simulink model "adaptive_dcmotor_2nd_sim"  (R2025b)
settings: Solver=FixedStepDiscrete  StartTime=0.0  StopTime=8  FixedStep=0.002  RelTol=1e-3
model workspace (MAT data in the model file):
  refProfile = [0 0.002 0.004 0.006 0.008 0.01 0.012 0.014 0.016 0.018 0.02 0.022 ... (8002 elements, 4001x2)]
(part 1 of 2)
settings Model: Creator=Lenard  LastModifiedBy=Lenard

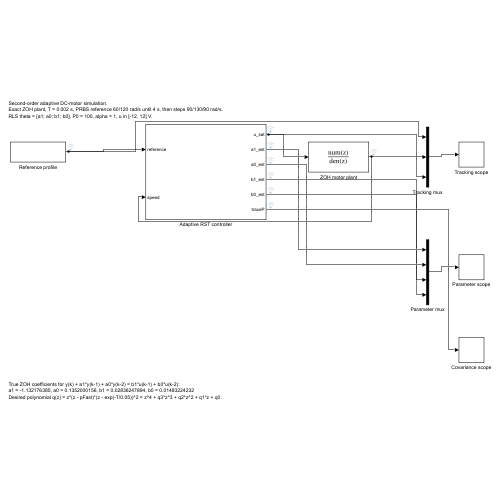
[thumbnail: Simulink's stored preview of the top-level diagram]
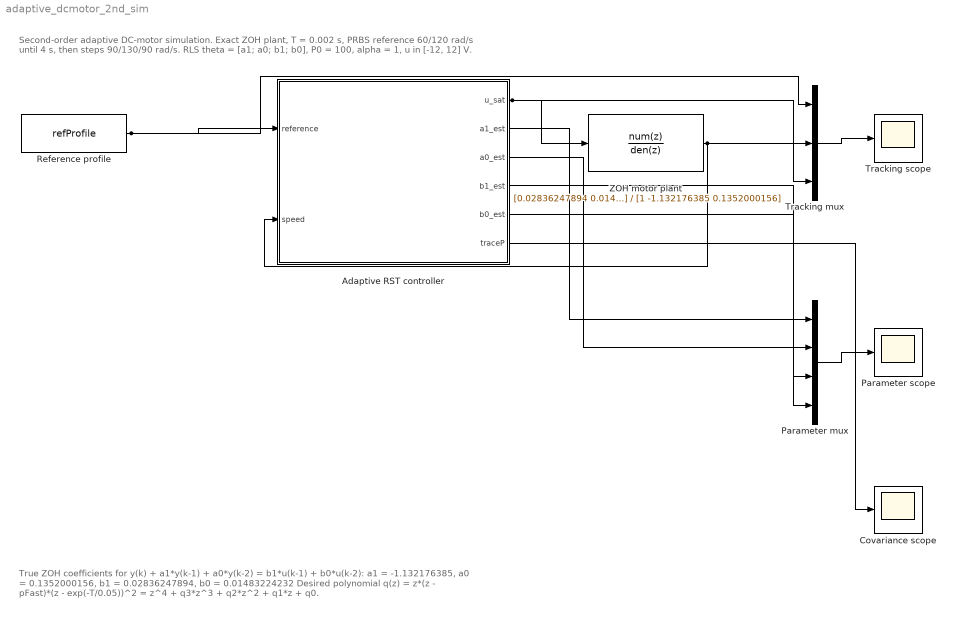
== system adaptive_dcmotor_2nd_sim ==
  note: Second-order adaptive DC-motor simulation.
      | Exact ZOH plant, T = 0.002 s, PRBS reference 60/120 rad/s until 4 s, then steps 90/130/90 rad/s.
      | RLS theta = [a1; a0; b1; b0], P0 = 100, alpha = 1, u in [-12, 12] V.
  note: True ZOH coefficients for y(k) + a1*y(k-1) + a0*y(k-2) = b1*u(k-1) + b0*u(k-2):
      | a1 = -1.132176385, a0 = 0.1352000156, b1 = 0.02836247894, b0 = 0.01483224232
      | Desired polynomial q(z) = z*(z - pFast)*(z - exp(-T/0.05))^2 = z^4 + q3*z^3 + q2*z^2 + q1*z + q0.
  Adaptive RST controller : Subsystem
  Covariance scope : Scope
  Parameter mux : Mux
  Parameter scope : Scope
  Reference profile : FromWorkspace  VariableName=refProfile  SampleTime=0.002  Interpolate=off  OutputAfterFinalValue=Holding final value
  Tracking mux : Mux  Inputs=3
  Tracking scope : Scope
  ZOH motor plant : DiscreteTransferFcn  Numerator=[0.02836247894 0.01483224232]  Denominator=[1 -1.132176385 0.1352000156]  SampleTime=0.002
  wires:
  Reference profile/1 -> Adaptive RST controller/1(reference), Tracking mux/1
  Adaptive RST controller/1(u_sat) -> ZOH motor plant/1, Tracking mux/3
  ZOH motor plant/1 -> Adaptive RST controller/2(speed), Tracking mux/2
  Tracking mux/1 -> Tracking scope/1
  Adaptive RST controller/2(a1_est) -> Parameter mux/1
  Adaptive RST controller/3(a0_est) -> Parameter mux/2
  Adaptive RST controller/4(b1_est) -> Parameter mux/3
  Adaptive RST controller/5(b0_est) -> Parameter mux/4
  Parameter mux/1 -> Parameter scope/1
  Adaptive RST controller/6(traceP) -> Covariance scope/1

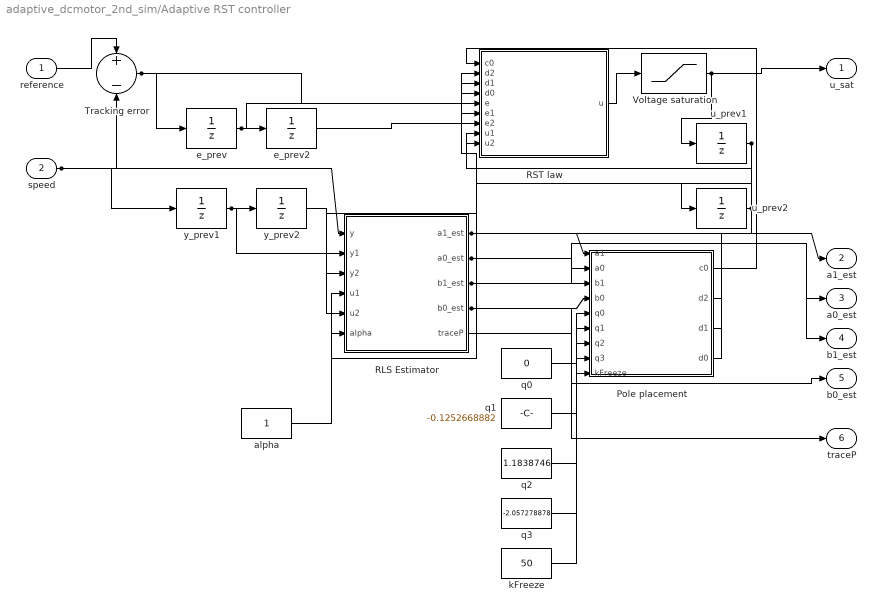
== system adaptive_dcmotor_2nd_sim/Adaptive RST controller ==
  reference : Inport
  speed : Inport  Port=2
  Pole placement : MATLAB Function  TreatAsAtomicUnit=on
  RLS Estimator : MATLAB Function  TreatAsAtomicUnit=on
  RST law : MATLAB Function  TreatAsAtomicUnit=on
  Tracking error : Sum  Inputs=+-
  Voltage saturation : Saturate  UpperLimit=12  LowerLimit=-12
  alpha : Constant
  e_prev : UnitDelay  SampleTime=0.002  HasFrameUpgradeWarning=on
  e_prev2 : UnitDelay  SampleTime=0.002  HasFrameUpgradeWarning=on
  kFreeze : Constant  Value=50
  q0 : Constant  Value=0
  q1 : Constant  Value=-0.1252668882
  q2 : Constant  Value=1.1838746
  q3 : Constant  Value=-2.057278878
  u_prev1 : UnitDelay  SampleTime=0.002  HasFrameUpgradeWarning=on
  u_prev2 : UnitDelay  SampleTime=0.002  HasFrameUpgradeWarning=on
  y_prev1 : UnitDelay  SampleTime=0.002  HasFrameUpgradeWarning=on
  y_prev2 : UnitDelay  SampleTime=0.002  HasFrameUpgradeWarning=on
  u_sat : Outport
  a1_est : Outport  Port=2
  a0_est : Outport  Port=3
  b1_est : Outport  Port=4
  b0_est : Outport  Port=5
  traceP : Outport  Port=6
  wires:
  reference/1 -> Tracking error/1
  speed/1 -> Tracking error/2, y_prev1/1, RLS Estimator/1(y)
  Tracking error/1 -> e_prev/1, RST law/5(e)
  e_prev/1 -> e_prev2/1, RST law/6(e1)
  e_prev2/1 -> RST law/7(e2)
  y_prev1/1 -> y_prev2/1, RLS Estimator/2(y1)
  y_prev2/1 -> RLS Estimator/3(y2)
  u_prev1/1 -> RLS Estimator/4(u1), RST law/8(u1), u_prev2/1
  u_prev2/1 -> RLS Estimator/5(u2), RST law/9(u2)
  alpha/1 -> RLS Estimator/6(alpha)
  RLS Estimator/1(a1_est) -> Pole placement/1(a1), a1_est/1
  RLS Estimator/2(a0_est) -> Pole placement/2(a0), a0_est/1
  RLS Estimator/3(b1_est) -> Pole placement/3(b1), b1_est/1
  RLS Estimator/4(b0_est) -> Pole placement/4(b0), b0_est/1
  q0/1 -> Pole placement/5(q0)
  q1/1 -> Pole placement/6(q1)
  q2/1 -> Pole placement/7(q2)
  q3/1 -> Pole placement/8(q3)
  kFreeze/1 -> Pole placement/9(kFreeze)
  Pole placement/1(c0) -> RST law/1(c0)
  Pole placement/2(d2) -> RST law/2(d2)
  Pole placement/3(d1) -> RST law/3(d1)
  Pole placement/4(d0) -> RST law/4(d0)
  RST law/1(u) -> Voltage saturation/1
  Voltage saturation/1 -> u_prev1/1, u_sat/1
  RLS Estimator/5(traceP) -> traceP/1
